simulink model "hw6_linear_pendulum"  (R2026a)
settings: Solver=ode4  StopTime=5  FixedStep=0.005
model workspace (MAT data in the model file):
  A = [0  1  0  0; 0  -0.181818181818  -2.67545454545  0; 0  0  0  1; 0  0.454545454545  31.2136363636  0]
  B = [0; 1.81818181818; 0; -4.54545454545]
  C = [1  0  0  0; 0  0  1  0]
  D = [0; 0]
settings Model: Creator=ievge  LastModifiedBy=ievge

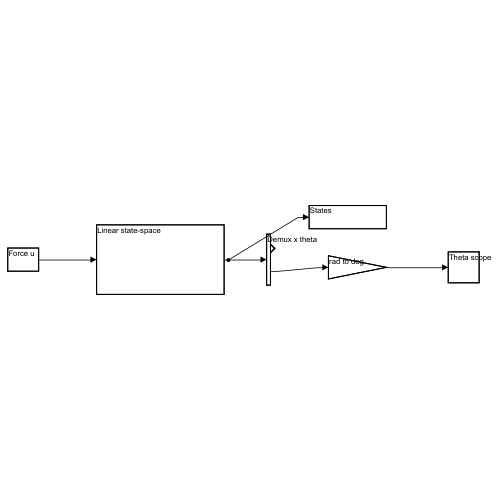
[thumbnail: Simulink's stored preview of the top-level diagram]
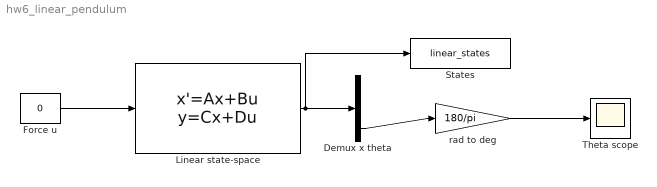
== system hw6_linear_pendulum ==
  Demux x theta : Demux  Outputs=2
  Force u : Constant  Value=0
  Linear state-space : StateSpace  A=A  B=B  C=C  D=D  InitialCondition=[0;0;10*pi/180;0]
  States : ToWorkspace  VariableName=linear_states  SaveFormat=Structure With Time  SampleTime=-1
  Theta scope : Scope
  rad to deg : Gain  Gain=180/pi
  wires:
  Force u/1 -> Linear state-space/1
  Linear state-space/1 -> Demux x theta/1, States/1
  Demux x theta/2 -> rad to deg/1
  rad to deg/1 -> Theta scope/1
